simulink model "veryfirstmodel"  (R2013a)
settings: Solver=ode4  StartTime=0.0  StopTime=1  FixedStep=1e-2  RelTol=1e-3
settings Model: Creator=ugurm  LastModifiedBy=ugurm

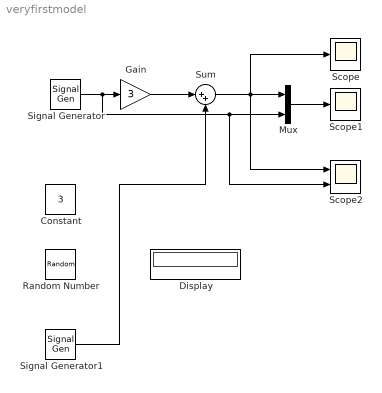
== system veryfirstmodel ==
  Constant : Constant  Value=3
  Display : Display
  Gain : Gain  Gain=3
  Mux : Mux  Inputs=2
  Random Number : RandomNumber  Variance=0.1  SampleTime=1e-2
  Scope : Scope
      settings: YMin=-10  YMax=10
  Scope1 : Scope
  Scope2 : Scope  NumInputPorts=2
      settings: YMin=-5~-5  YMax=5~5  SaveName=ScopeData2
  Signal Generator : SignalGenerator  Frequency=50
  Signal Generator1 : SignalGenerator  Amplitude=0.4  Frequency=150
  Sum : Sum  Inputs=|++
  wires:
  Signal Generator/1 -> Scope2/2, Mux/2, Gain/1
  Gain/1 -> Sum/1
  Signal Generator1/1 -> Sum/2
  Sum/1 -> Scope2/1, Mux/1, Scope/1
  Mux/1 -> Scope1/1
